simulink model "zad2wariant1"  (R2023a)
settings: Solver=VariableStepAuto  StartTime=0.0  StopTime=30  RelTol=1e-3
values from neighbouring files (symbols this model uses):
  a1 = Gz.Numerator{1}(2)    [zad1.m]
  a2 = Gz.Numerator{1}(3)    [zad1.m]
  a3 = Gz.Numerator{1}(4)    [zad1.m]
  b1 = Gz.Denominator{1}(2)    [zad1.m]
  b2 = Gz.Denominator{1}(3)    [zad1.m]
  b3 = Gz.Denominator{1}(4)    [zad1.m]
  T = 0.5    [zad1.m]
settings Model: Creator=pkutyl  LastModifiedBy=denys

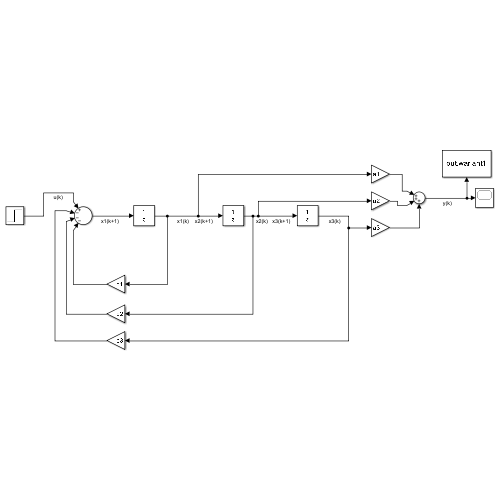
[thumbnail: Simulink's stored preview of the top-level diagram]
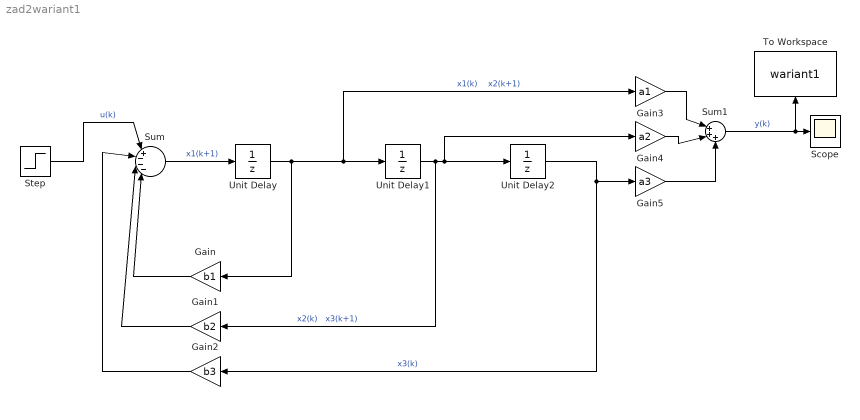
== system zad2wariant1 ==
  Gain : Gain  Gain=b1
  Gain1 : Gain  Gain=b2
  Gain2 : Gain  Gain=b3
  Gain3 : Gain  Gain=a1
  Gain4 : Gain  Gain=a2
  Gain5 : Gain  Gain=a3
  Scope : Scope
  Step : Step  SampleTime=T
  Sum : Sum  Inputs=|+---|
  Sum1 : Sum  Inputs=|+++
  To Workspace : ToWorkspace  VariableName=wariant1  SaveFormat=Timeseries  SampleTime=T
  Unit Delay : UnitDelay  SampleTime=-1  HasFrameUpgradeWarning=on
  Unit Delay1 : UnitDelay  SampleTime=-1  HasFrameUpgradeWarning=on
  Unit Delay2 : UnitDelay  SampleTime=-1  HasFrameUpgradeWarning=on
  wires:
  Step/1 -> Sum/1  "u(k)"
  Sum/1 -> Unit Delay/1  "x1(k+1)"
  Unit Delay/1 -> Gain3/1, Unit Delay1/1, Gain/1  "x1(k)    x2(k+1)"
  Unit Delay1/1 -> Unit Delay2/1, Gain4/1, Gain1/1  "x2(k)   x3(k+1)"
  Unit Delay2/1 -> Gain2/1, Gain5/1  "x3(k)"
  Sum1/1 -> Scope/1, To Workspace/1  "y(k)"
  Gain/1 -> Sum/4
  Gain1/1 -> Sum/3
  Gain2/1 -> Sum/2
  Gain3/1 -> Sum1/1
  Gain4/1 -> Sum1/2
  Gain5/1 -> Sum1/3
